simulink model "fig7_45"  (Simulink 6.1)
settings: Solver=ode45  StartTime=0.0  StopTime=100.0  RelTol=1e-3
values from neighbouring files (symbols this model uses):
  cc = K    [fig10_21.m]    (also in fig10_22.m; fig10_23.m; fig10_24.m)
undefined symbols (not defined in the file or in its folder): aa, bb, dd
libraries: simulink x1
settings Model: LastModifiedBy=abbas  ExtModeTrigMode=oneshot  ExtModeArmWhenConnect=off
settings DataIOCC: LimitDataPoints=off
settings OptimizationCC: BlockReduction=off  BooleanDataType=off
settings HardwareCC: TargetUnknown=on
settings STFCustomTargetCC: TargetFcnLib=ansi_tfl_tmw.mat  GenFloatMathFcnCalls=ANSI_C  ModelReferenceCompliant=off  SystemTargetFile=grt.tlc

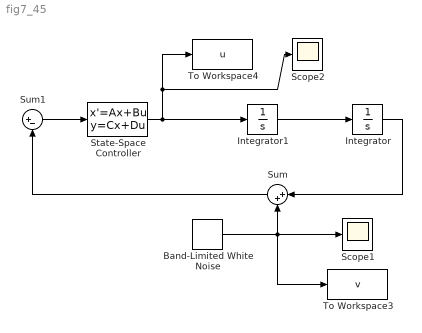
== system fig7_45 ==
  Band-Limited White Noise : simulink/Sources/Band-Limited White Noise  Cov=[0.1]  Ts=0.05  seed=[23341]
  Integrator : Integrator
  Integrator1 : Integrator
  Scope1 : Scope
      settings: YMin=-12.5  YMax=10
  Scope2 : Scope
      settings: YMin=-12.5  YMax=10
  State-Space Controller : StateSpace  A=aa  B=bb  C=cc  D=dd
  Sum : Sum  Orientation=left  Inputs=|++  SaturateOnIntegerOverflow=on  InputSameDT=on
  Sum1 : Sum  Inputs=|+-  SaturateOnIntegerOverflow=on  InputSameDT=on
  To Workspace3 : ToWorkspace  VariableName=v  SampleTime=0.0  SaveFormat=Array
  To Workspace4 : ToWorkspace  VariableName=u  SampleTime=0.0  SaveFormat=Array
  wires:
  Integrator1/1 -> Integrator/1
  Integrator/1 -> Sum/1
  Sum/1 -> Sum1/2
  Sum1/1 -> State-Space Controller/1
  Band-Limited White Noise/1 -> Sum/2, Scope1/1, To Workspace3/1
  State-Space Controller/1 -> Integrator1/1, To Workspace4/1, Scope2/1
